simulink model "RELY_PT_Simscape_model_clean"  (R2023b)
settings: Solver=VariableStepAuto  StartTime=0.0  StopTime=90  RelTol=1e-3
PreLoadFcn:
  | %warning('off', 'physmod:simscape:engine:sli:zc:ZeroCrossingsGloballyOff');
  | %warning('off', 'SimulinkExecution:DE:MinStepSizeForDAEWarning');
  | %warning('off')
StopFcn:
  | [lastWarningMessage, warningId] = lastwarn
  | display(lastwarn)
model workspace (MAT data in the model file):
  H_n0_a0 = 0
  H_n0_a12 = 0
  H_n0_a18 = 0
  H_n0_a24 = 0
  H_n0_a3 = 0
  H_n0_a30 = 0
  H_n0_a6 = 0
  H_n1000_a0 = 41.890778
  H_n1000_a12 = [39.720451 39.531112 38.954187 38.409379 37.371519 36.969249 36.145323 35.016504 34.41791 32.725714 29.62353 26.475564 ... (14 elements, 14x1)]
  H_n1000_a18 = [40.963701 39.338792 38.382958 37.856819 36.842644 36.842643 36.420949 35.987956 35.163037 34.563355 33.765342 32.552991 ... (15 elements, 15x1)]
  H_n1000_a24 = [38.981139 38.080649 37.518525 37.024422 36.538756 36.021688 35.445183 35.316271 34.435388 33.472576 31.549447 29.78877 ... (14 elements, 14x1)]
  H_n1000_a3 = [41.890778; 40.628119; 36.670096; 26.463116; 15.07804; 14.630001]
  H_n1000_a30 = [38.909304 37.733775 37.005538 36.587968 36.205827 35.762706 35.340739 35.100753 34.52749 33.838404 32.675216 31.34989 ... (15 elements, 15x1)]
  H_n1000_a6 = [40.993428; 40.166943; 39.662948; 38.765772; 36.424758; 29.65575; 24.303713; 16.252806]
  H_n200_a0 = 3.238104
  H_n200_a12 = [1.067777; 1.033602; 0.921547; 0.765236; 0.326687]
  H_n200_a18 = [2.311027; 0.686118; 0]
  H_n200_a24 = [0.328465; 0]
  H_n200_a3 = [3.238104; 1.975445; 0]
  H_n200_a30 = [0.25663; 0]
  H_n200_a6 = [2.340754; 1.514269; 1.010274; 0.113098; 0]
  H_n300_a0 = 5.257449
  H_n300_a12 = [3.087122; 2.979731; 2.862074; 2.645072; 2.104165; 1.313568; 0.689971; 0.506891]
  H_n300_a18 = [4.330372; 2.705463; 1.749629; 1.22349; 0.209315; 0.209314; 0]
  H_n300_a24 = [2.34781; 1.44732; 0.885196; 0.391093; 0]
  H_n300_a3 = [5.257449; 3.99479; 0.036767; 0]
  H_n300_a30 = [2.275975; 1.100446; 0.372209; 0]
  H_n300_a6 = [4.360099; 3.533614; 3.029619; 2.132443; 0]
  H_n400_a0 = 8.103137
  H_n400_a12 = [5.93281; 5.819804; 5.646321; 5.369927; 5.096687; 4.506441; 3.638024; 2.520335; 1.315366]
  H_n400_a18 = [7.17606; 5.551151; 4.595317; 4.069178; 3.055003; 3.055002; 2.633308; 2.200315; 1.375396; 0.775714; 0]
  H_n400_a24 = [5.193498; 4.293008; 3.730884; 3.236781; 2.751115; 2.234047; 1.657542; 1.52863; 0.647747; 0]
  H_n400_a3 = [8.103137; 6.840478; 2.882455; 0]
  H_n400_a30 = [5.121663; 3.946134; 3.217897; 2.800327; 2.418186; 1.975065; 1.553098; 1.313112; 0.739849; 0.050763; 0]
  H_n400_a6 = [7.205787; 6.379302; 5.875307; 4.978131; 2.637117; 0]
  H_n500_a0 = 11.717619
  H_n500_a12 = [9.547292; 9.47316; 9.245124; 8.930514; 8.600563; 8.213538; 7.488479; 5.941616; 4.256148; 2.697226; 2.352739]
  H_n500_a18 = [10.790542 9.165633 8.209799 7.68366 6.669485 6.669484 6.24779 5.814797 4.989878 4.390196 3.592183 2.379832 ... (14 elements, 14x1)]
  H_n500_a24 = [8.80798; 7.90749; 7.345366; 6.851263; 6.365597; 5.848529; 5.272024; 5.143112; 4.262229; 3.299417; 1.376288; 0]
  H_n500_a3 = [11.717619; 10.45496; 6.496937; 0]
  H_n500_a30 = [8.736145 7.560616 6.832379 6.414809 6.032668 5.589547 5.16758 4.927594 4.354331 3.665245 2.502057 1.176731 ... (13 elements, 13x1)]
  H_n500_a6 = [10.820269; 9.993784; 9.489789; 8.592613; 6.251599; 0]
  H_n600_a0 = 16.132839
  H_n600_a12 = [13.962512; 13.826181; 13.39772; 12.968961; 12.407512; 11.706692; 10.267649; 7.799717; 4.805174; 3.660927]
  H_n600_a18 = [15.205762 13.580853 12.625019 12.09888 11.084705 11.084704 10.66301 10.230017 9.405098 8.805416 8.007403 6.795052 ... (15 elements, 15x1)]
  H_n600_a24 = [13.2232 12.32271 11.760586 11.266483 10.780817 10.263749 9.687244 9.558332 8.677449 7.714637 5.791508 4.030831 ... (14 elements, 14x1)]
  H_n600_a3 = [16.132839; 14.87018; 10.912157; 0.705177; 0]
  H_n600_a30 = [13.151365 11.975836 11.247599 10.830029 10.447888 10.004767 9.5828 9.342814 8.769551 8.080465 6.917277 5.591951 ... (15 elements, 15x1)]
  H_n600_a6 = [15.235489; 14.409004; 13.905009; 13.007833; 10.666819; 3.897811; 0]
  H_n800_a0 = 27.361581
  H_n800_a12 = [25.191254 25.111402 24.820598 24.424515 23.864287 23.409359 22.670967 21.888411 20.849925 19.271611 15.931711 12.191149 ... (13 elements, 13x1)]
  H_n800_a18 = [26.434504 24.809595 23.853761 23.327622 22.313447 22.313446 21.891752 21.458759 20.63384 20.034158 19.236145 18.023794 ... (15 elements, 15x1)]
  H_n800_a24 = [24.451942 23.551452 22.989328 22.495225 22.009559 21.492491 20.915986 20.787074 19.906191 18.943379 17.02025 15.259573 ... (14 elements, 14x1)]
  H_n800_a3 = [27.361581; 26.098922; 22.140899; 11.933919; 0.548843; 0.100804]
  H_n800_a30 = [24.380107 23.204578 22.476341 22.058771 21.67663 21.233509 20.811542 20.571556 19.998293 19.309207 18.146019 16.820693 ... (15 elements, 15x1)]
  H_n800_a6 = [26.464231; 25.637746; 25.133751; 24.236575; 21.895561; 15.126553; 9.774516; 1.723609]
  Q_n0_a0 = 0
  Q_n0_a12 = 0
  Q_n0_a18 = 0
  Q_n0_a24 = 0
  Q_n0_a3 = 0
  Q_n0_a30 = 0
  Q_n0_a6 = 0
  Q_n1000_a0 = 0
  Q_n1000_a12 = [1.414248 19.568281 42.238315 63.498226 84.388459 102.222447 118.464783 143.286635 161.301465 179.936079 204.714875 220.907445 ... (14 elements, 14x1)]
  Q_n1000_a18 = [1.408805 18.494853 42.193847 62.613149 82.187881 100.830014 121.754975 143.135578 163.193197 178.395322 191.000248 206.658481 ... (15 elements, 15x1)]
  Q_n1000_a24 = [1.423901 19.712366 41.694896 61.712178 79.84989 98.707828 119.980398 158.480134 182.365548 200.814664 230.378522 251.54405 ... (14 elements, 14x1)]
  Q_n1000_a3 = [1.421904; 19.241198; 41.163866; 59.088119; 65.74439; 65.877885]
  Q_n1000_a30 = [1.416544 19.140809 40.908666 60.206263 78.832144 103.65752 124.537322 147.320333 173.202338 192.924112 213.836687 234.126658 ... (15 elements, 15x1)]
  Q_n1000_a6 = [1.391187; 19.624304; 38.811559; 58.375933; 80.275679; 102.989156; 113.538726; 121.386064]
  Q_n200_a0 = 0
  Q_n200_a12 = [1.34007; 7.497876; 25.362531; 37.225803; 48.080824]
  Q_n200_a18 = [1.408805; 18.494853; 42.193847]
  Q_n200_a24 = [1.423901; 19.712366]
  Q_n200_a3 = [1.421904; 19.241198; 41.163866]
  Q_n200_a30 = [1.416544; 19.140809]
  Q_n200_a6 = [1.391187; 19.624304; 38.811559; 58.375933; 80.275679]
  Q_n300_a0 = 0
  Q_n300_a12 = [1.367844; 15.571876; 31.1207; 46.669706; 61.781875; 72.981285; 80.669073; 83.063222]
  Q_n300_a18 = [1.408805; 18.494853; 42.193847; 62.613149; 82.187881; 100.830014; 121.754975]
  Q_n300_a24 = [1.423901; 19.712366; 41.694896; 61.712178; 79.84989]
  Q_n300_a3 = [1.421904; 19.241198; 41.163866; 59.088119]
  Q_n300_a30 = [1.416544; 19.140809; 40.908666; 60.206263]
  Q_n300_a6 = [1.391187; 19.624304; 38.811559; 58.375933; 80.275679]
  Q_n400_a0 = 0
  Q_n400_a12 = [1.344743; 14.017933; 27.304134; 46.234876; 61.473368; 76.555174; 87.737013; 99.497539; 110.117964]
  Q_n400_a18 = [1.408805; 18.494853; 42.193847; 62.613149; 82.187881; 100.830014; 121.754975; 143.135578; 163.193197; 178.395322; 191.000248]
  Q_n400_a24 = [1.423901; 19.712366; 41.694896; 61.712178; 79.84989; 98.707828; 119.980398; 158.480134; 182.365548; 200.814664]
  Q_n400_a3 = [1.421904; 19.241198; 41.163866; 59.088119]
  Q_n400_a30 = [1.416544; 19.140809; 40.908666; 60.206263; 78.832144; 103.65752; 124.537322; 147.320333; 173.202338; 192.924112; 213.836687]
  Q_n400_a6 = [1.391187; 19.624304; 38.811559; 58.375933; 80.275679; 102.989156]
  Q_n500_a0 = 0
  Q_n500_a12 = [1.413707; 13.380401; 28.647003; 44.528782; 60.801181; 80.900847; 92.946609; 109.551251; 123.738046; 134.385391; 136.883854]
  Q_n500_a18 = [1.408805 18.494853 42.193847 62.613149 82.187881 100.830014 121.754975 143.135578 163.193197 178.395322 191.000248 206.658481 ... (14 elements, 14x1)]
  Q_n500_a24 = [1.423901; 19.712366; 41.694896; 61.712178; 79.84989; 98.707828; 119.980398; 158.480134; 182.365548; 200.814664; 230.378522; 251.54405]
  Q_n500_a3 = [1.421904; 19.241198; 41.163866; 59.088119]
  Q_n500_a30 = [1.416544 19.140809 40.908666 60.206263 78.832144 103.65752 124.537322 147.320333 173.202338 192.924112 213.836687 234.126658 ... (13 elements, 13x1)]
  Q_n500_a6 = [1.391187; 19.624304; 38.811559; 58.375933; 80.275679; 102.989156]
  Q_n600_a0 = 0
  Q_n600_a12 = [1.382688; 19.531879; 40.922311; 61.362127; 81.302459; 103.019269; 120.607387; 139.781266; 159.674546; 165.725558]
  Q_n600_a18 = [1.408805 18.494853 42.193847 62.613149 82.187881 100.830014 121.754975 143.135578 163.193197 178.395322 191.000248 206.658481 ... (15 elements, 15x1)]
  Q_n600_a24 = [1.423901 19.712366 41.694896 61.712178 79.84989 98.707828 119.980398 158.480134 182.365548 200.814664 230.378522 251.54405 ... (14 elements, 14x1)]
  Q_n600_a3 = [1.421904; 19.241198; 41.163866; 59.088119; 65.74439]
  Q_n600_a30 = [1.416544 19.140809 40.908666 60.206263 78.832144 103.65752 124.537322 147.320333 173.202338 192.924112 213.836687 234.126658 ... (15 elements, 15x1)]
  Q_n600_a6 = [1.391187; 19.624304; 38.811559; 58.375933; 80.275679; 102.989156; 113.538726]
  Q_n800_a0 = 0
  Q_n800_a12 = [1.454137 13.240478 29.958658 46.304107 64.130487 81.966165 101.000644 121.860549 141.622312 158.000863 181.468089 200.017812 ... (13 elements, 13x1)]
  Q_n800_a18 = [1.408805 18.494853 42.193847 62.613149 82.187881 100.830014 121.754975 143.135578 163.193197 178.395322 191.000248 206.658481 ... (15 elements, 15x1)]
  Q_n800_a24 = [1.423901 19.712366 41.694896 61.712178 79.84989 98.707828 119.980398 158.480134 182.365548 200.814664 230.378522 251.54405 ... (14 elements, 14x1)]
  Q_n800_a3 = [1.421904; 19.241198; 41.163866; 59.088119; 65.74439; 65.877885]
  Q_n800_a30 = [1.416544 19.140809 40.908666 60.206263 78.832144 103.65752 124.537322 147.320333 173.202338 192.924112 213.836687 234.126658 ... (15 elements, 15x1)]
  Q_n800_a6 = [1.391187; 19.624304; 38.811559; 58.375933; 80.275679; 102.989156; 113.538726; 121.386064]
  Qt_n0_a0 = 0
  Qt_n0_a12 = 0
  Qt_n0_a18 = 0
  Qt_n0_a24 = 0
  Qt_n0_a3 = 0
  Qt_n0_a30 = 0
  Qt_n0_a6 = 0
  Qt_n1000_a0 = 0
  Qt_n1000_a12 = [0 16.7063426923 33.4126853846 50.1190280769 66.8253707692 83.5317134615 100.238056154 116.944398846 133.650741538 150.357084231 167.063426923 183.769769615 ... (14 elements, 14x1)]
  Qt_n1000_a18 = [0 19.1696658462 38.3393316923 57.5089975385 76.6786633846 95.8483292308 115.017995077 134.187660923 153.357326769 172.526992615 191.696658462 210.866324308 ... (14 elements, 14x1)]
  Qt_n1000_a24 = [0 21.8796540769 43.7593081538 65.6389622308 87.5186163077 109.398270385 131.277924462 153.157578538 175.037232615 196.916886692 218.796540769 240.676194846 ... (14 elements, 14x1)]
  Qt_n1000_a3 = [0 5.06752961538 10.1350592308 15.2025888462 20.2701184615 25.3376480769 30.4051776923 35.4727073077 40.5402369231 45.6077665385 50.6752961538 55.7428257692 ... (14 elements, 14x1)]
  Qt_n1000_a30 = [0 22.2052569231 44.4105138462 66.6157707692 88.8210276923 111.026284615 133.231541538 155.436798462 177.642055385 199.847312308 222.052569231 244.257826154 ... (14 elements, 14x1)]
  Qt_n1000_a6 = [0 9.33738953846 18.6747790769 28.0121686154 37.3495581538 46.6869476923 56.0243372308 65.3617267692 74.6991163077 84.0365058462 93.3738953846 102.711284923 ... (14 elements, 14x1)]
  Qt_n200_a0 = 0
  Qt_n200_a12 = [0; 54.29561375; 108.5912275; 162.88684125; 217.182455]
  Qt_n200_a18 = [0; 62.301414; 124.602828; 186.904242; 249.205656]
  Qt_n200_a24 = [0; 71.10887575; 142.2177515; 213.32662725; 284.435503]
  Qt_n200_a3 = [0; 16.46947125; 32.9389425; 49.40841375; 65.877885]
  Qt_n200_a30 = [0; 72.167085; 144.33417; 216.501255; 288.66834]
  Qt_n200_a6 = [0; 30.346516; 60.693032; 91.039548; 121.386064]
  Qt_n300_a0 = 0
  Qt_n300_a12 = [0; 31.026065; 62.05213; 93.078195; 124.10426; 155.130325; 186.15639; 217.182455]
  Qt_n300_a18 = [0; 35.600808; 71.201616; 106.802424; 142.403232; 178.00404; 213.604848; 249.205656]
  Qt_n300_a24 = [0; 40.6336432857; 81.2672865714; 121.900929857; 162.534573143; 203.168216429; 243.801859714; 284.435503]
  Qt_n300_a3 = [0; 9.41112642857; 18.8222528571; 28.2333792857; 37.6445057143; 47.0556321429; 56.4667585714; 65.877885]
  Qt_n300_a30 = [0; 41.2383342857; 82.4766685714; 123.715002857; 164.953337143; 206.191671429; 247.430005714; 288.66834]
  Qt_n300_a6 = [0; 17.3408662857; 34.6817325714; 52.0225988571; 69.3634651429; 86.7043314286; 104.045197714; 121.386064]
  Qt_n400_a0 = 0
  Qt_n400_a12 = [0; 27.147806875; 54.29561375; 81.443420625; 108.5912275; 135.739034375; 162.88684125; 190.034648125; 217.182455]
  Qt_n400_a18 = [0; 31.150707; 62.301414; 93.452121; 124.602828; 155.753535; 186.904242; 218.054949; 249.205656]
  Qt_n400_a24 = [0; 35.554437875; 71.10887575; 106.663313625; 142.2177515; 177.772189375; 213.32662725; 248.881065125; 284.435503]
  Qt_n400_a3 = [0; 8.234735625; 16.46947125; 24.704206875; 32.9389425; 41.173678125; 49.40841375; 57.643149375; 65.877885]
  Qt_n400_a30 = [0; 36.0835425; 72.167085; 108.2506275; 144.33417; 180.4177125; 216.501255; 252.5847975; 288.66834]
  Qt_n400_a6 = [0; 15.173258; 30.346516; 45.519774; 60.693032; 75.86629; 91.039548; 106.212806; 121.386064]
  Qt_n500_a0 = 0
  Qt_n500_a12 = [0; 21.7182455; 43.436491; 65.1547365; 86.872982; 108.5912275; 130.309473; 152.0277185; 173.745964; 195.4642095; 217.182455]
  Qt_n500_a18 = [0; 24.9205656; 49.8411312; 74.7616968; 99.6822624; 124.602828; 149.5233936; 174.4439592; 199.3645248; 224.2850904; 249.205656]
  Qt_n500_a24 = [0; 28.4435503; 56.8871006; 85.3306509; 113.7742012; 142.2177515; 170.6613018; 199.1048521; 227.5484024; 255.9919527; 284.435503]
  Qt_n500_a3 = [0; 6.5877885; 13.175577; 19.7633655; 26.351154; 32.9389425; 39.526731; 46.1145195; 52.702308; 59.2900965; 65.877885]
  Qt_n500_a30 = [0; 28.866834; 57.733668; 86.600502; 115.467336; 144.33417; 173.201004; 202.067838; 230.934672; 259.801506; 288.66834]
  Qt_n500_a6 = [0; 12.1386064; 24.2772128; 36.4158192; 48.5544256; 60.693032; 72.8316384; 84.9702448; 97.1088512; 109.2474576; 121.386064]
  Qt_n600_a0 = 0
  Qt_n600_a12 = [0; 24.1313838889; 48.2627677778; 72.3941516667; 96.5255355556; 120.656919444; 144.788303333; 168.919687222; 193.051071111; 217.182455]
  Qt_n600_a18 = [0; 27.6895173333; 55.3790346667; 83.068552; 110.758069333; 138.447586667; 166.137104; 193.826621333; 221.516138667; 249.205656]
  Qt_n600_a24 = [0; 31.6039447778; 63.2078895556; 94.8118343333; 126.415779111; 158.019723889; 189.623668667; 221.227613444; 252.831558222; 284.435503]
  Qt_n600_a3 = [0; 7.319765; 14.63953; 21.959295; 29.27906; 36.598825; 43.91859; 51.238355; 58.55812; 65.877885]
  Qt_n600_a30 = [0; 32.07426; 64.14852; 96.22278; 128.29704; 160.3713; 192.44556; 224.51982; 256.59408; 288.66834]
  Qt_n600_a6 = [0; 13.4873404444; 26.9746808889; 40.4620213333; 53.9493617778; 67.4367022222; 80.9240426667; 94.4113831111; 107.898723556; 121.386064]
  Qt_n800_a0 = 0
  Qt_n800_a12 = [1.454137 13.240478 29.958658 46.304107 64.130487 81.966165 101.000644 121.860549 141.622312 158.000863 181.468089 200.017812 ... (13 elements, 13x1)]
  Qt_n800_a18 = [1.408805 18.494853 42.193847 62.613149 82.187881 100.830014 121.754975 143.135578 163.193197 178.395322 191.000248 206.658481 ... (15 elements, 15x1)]
  Qt_n800_a24 = [1.423901 19.712366 41.694896 61.712178 79.84989 98.707828 119.980398 158.480134 182.365548 200.814664 230.378522 251.54405 ... (14 elements, 14x1)]
  Qt_n800_a3 = [1.421904; 19.241198; 41.163866; 59.088119; 65.74439; 65.877885]
  Qt_n800_a30 = [1.416544 19.140809 40.908666 60.206263 78.832144 103.65752 124.537322 147.320333 173.202338 192.924112 213.836687 234.126658 ... (15 elements, 15x1)]
  Qt_n800_a6 = [1.391187; 19.624304; 38.811559; 58.375933; 80.275679; 102.989156; 113.538726; 121.386064]
  T_n0_a0 = 0
  T_n0_a12 = 0
  T_n0_a18 = 0
  T_n0_a24 = 0
  T_n0_a3 = 0
  T_n0_a30 = 0
  T_n0_a6 = 0
  T_n1000_a0 = 212.918607715
  T_n1000_a12 = [277.00328 303.197846 359.332799 415.990553 473.006501 524.971962 568.439998 614.751636 645.453671 686.416528 736.459699 766.00495 ... (14 elements, 14x1)]
  T_n1000_a18 = [404.787518585 404.787519585 404.787520585 452.001035443 510.769182758 569.170823248 619.258390544 671.193440572 702.288039208 740.090455903 784.6835679 804.130666851 ... (14 elements, 14x1)]
  T_n1000_a24 = [392.733848002 392.733849002 439.832412682 496.757162262 558.754412487 616.785919809 664.650726048 714.600674645 742.820149063 778.056363106 818.81453792 829.567277535 ... (14 elements, 14x1)]
  T_n1000_a3 = [212.918607715 212.918608715 228.059187273 245.258629322 263.444651993 280.537619561 295.489881395 314.864010802 328.777823048 350.303733023 379.296474597 399.333660461 ... (14 elements, 14x1)]
  T_n1000_a30 = [421.41608902 421.41609002 440.120958305 494.847705165 558.496053897 619.777761537 670.689767338 722.468413619 750.521719432 783.871432441 821.31664772 828.125692716 ... (14 elements, 14x1)]
  T_n1000_a6 = [230.781502838 242.11861906 275.591838884 308.353632665 342.191487589 374.384720871 403.309826474 437.782449643 463.92378222 499.743176352 544.837963229 574.949829916 ... (14 elements, 14x1)]
  T_n200_a0 = 11.7025560582
  T_n200_a12 = [15.224815; 17.437209; 27.286419; 32.75526; 36.736891]
  T_n200_a18 = [22.2481664649; 22.2481674649; 29.7967404674; 35.0029856064; 37.9298346396]
  T_n200_a24 = [21.5856656285; 21.5856666285; 31.8450559685; 36.603000066; 37.244980588]
  T_n200_a3 = [11.7025560582; 11.7025570582; 14.0701061615; 16.8185305371; 19.8004114128]
  T_n200_a30 = [23.1621156015; 23.1621166015; 32.1752703252; 36.7584990128; 37.0567955811]
  T_n200_a6 = [12.6843468645; 12.8324608472; 19.3918858683; 24.1271526112; 28.1688483977]
  T_n300_a0 = 21.9563918625
  T_n300_a12 = [28.564871; 37.811393; 51.060297; 62.173487; 71.550804; 76.450124; 78.444822; 79.17734]
  T_n300_a18 = [41.7421167388; 42.9108918828; 55.1360860791; 67.6540960449; 78.0129967452; 82.131335262; 82.2106920633; 82.2106930633]
  T_n300_a24 = [40.4991294887; 46.5570500429; 60.4440800927; 72.9025088968; 82.8132330772; 86.1815876807; 86.1815886807; 86.1815896807]
  T_n300_a3 = [21.9563918625; 24.2987024018; 28.8525912211; 32.6741136324; 36.5007981988; 39.0750608961; 40.992116131; 42.6749206015]
  T_n300_a30 = [43.4568724969; 46.6716879727; 60.3340767989; 73.4500908753; 83.7275835225; 86.7267109875; 86.7267119875; 86.7267129875]
  T_n300_a6 = [23.798432487; 29.1774180928; 37.1526626527; 44.1911964018; 51.0954995027; 55.8783235655; 59.0146995211; 60.7110298744]
  T_n400_a0 = 36.5747783831
  T_n400_a12 = [47.583129; 57.587133; 70.997483; 92.596133; 105.648342; 118.067856; 125.504464; 132.006944; 135.802681]
  T_n400_a18 = [69.533677415; 69.533678415; 76.8740175836; 100.303252833; 115.367876869; 128.336169471; 134.116808932; 137.955920328; 140.212551845]
  T_n400_a24 = [67.4631193976; 71.5608625438; 84.4618055352; 108.830263209; 123.298603747; 135.640440023; 140.247395505; 141.469481676; 141.469482676]
  T_n400_a3 = [36.5747783831; 37.7251893206; 41.1960296213; 49.6890098491; 54.4770417739; 60.123752896; 64.4415785534; 69.2427899981; 73.1947881697]
  T_n400_a30 = [72.390103563; 72.390104563; 84.1709945503; 109.287902187; 124.577137193; 137.012881865; 140.843202467; 141.001174713; 141.001175713]
  T_n400_a6 = [39.6432346229; 44.8168070482; 52.2487527018; 66.1049603064; 75.082061528; 84.972188629; 92.4451631986; 99.6500611017; 104.129800562]
  T_n500_a0 = 54.638111826
  T_n500_a12 = [71.083201; 82.173064; 102.133248; 124.085102; 147.054333; 166.819409; 179.223177; 194.174843; 204.809839; 209.250296; 210.496478]
  T_n500_a18 = [103.874555369; 103.874556369; 111.971411057; 133.975134134; 159.674103654; 182.16661684; 195.237724451; 209.113945989; 216.990100397; 217.817160263; 217.817161263]
  T_n500_a24 = [100.781402506; 103.745756337; 122.884743199; 146.67783451; 172.687108198; 194.6892854; 206.759491412; 219.699188786; 225.542233105; 225.542234105; 225.542235105]
  T_n500_a3 = [54.638111826; 55.3756440027; 61.8869149757; 69.4496573087; 78.1013520092; 86.0195980434; 91.3358717102; 99.1482056914; 105.978124691; 110.324399881; 113.453173415]
  T_n500_a30 = [108.14169623; 108.14169723; 122.461015878; 146.537256202; 173.69605955; 196.708097903; 208.970369715; 221.255795744; 225.791005625; 225.791006625; 225.791007625]
  T_n500_a6 = [59.2219989356; 64.7472437047; 76.6568548901; 89.9397391904; 104.73390719; 118.55505627; 128.538611573; 141.568983951; 152.461177958; 158.612181364; 161.402971662]
  T_n600_a0 = 76.867003996
  T_n600_a12 = [100.00259; 121.04164; 155.003179; 190.565914; 219.357637; 243.674297; 266.051748; 283.258948; 297.465728; 299.083675]
  T_n600_a18 = [146.134732622; 146.134733622; 168.784930149; 205.972762496; 238.873142197; 265.77258359; 287.747983451; 301.365627068; 310.186180583; 310.186181583]
  T_n600_a24 = [141.78316582; 151.644017044; 185.472115884; 224.665102596; 256.903171302; 282.518160305; 303.137003848; 314.154023247; 317.032846233; 317.032847233]
  T_n600_a3 = [76.867003996; 80.5184824525; 92.0750202273; 104.524650538; 114.657143003; 124.465033252; 135.526566037; 146.079378975; 156.481270539; 161.199808984]
  T_n600_a30 = [152.137911037; 153.157263195; 184.752954542; 224.955132121; 259.040760261; 285.649929708; 305.759721542; 314.944478723; 315.773465036; 315.773466036]
  T_n600_a6 = [83.3157932567; 94.825703277; 115.297380604; 137.074433445; 155.769374031; 173.678780092; 192.721213139; 209.938294249; 225.088940119; 229.32922384]
  T_n800_a0 = 134.014292
  T_n800_a12 = [177.472657 191.031966 222.274404 256.025382 295.517459 337.418928 374.986676 405.355521 436.442001 464.646182 498.675007 515.239787 ... (13 elements, 13x1)]
  T_n800_a18 = [258.973744 258.973745 261.725534 300.744533 341.164912 384.371738 411.583185 443.99362 474.009937 494.394349 508.380623 522.912901 ... (15 elements, 15x1)]
  T_n800_a24 = [249.324679 250.177033 276.500869 309.026906 346.334209 381.490782 412.86896 468.224431 499.703761 515.781407 537.873966 541.192558 ... (14 elements, 14x1)]
  T_n800_a3 = [134.014292; 165.189551; 220.071093; 267.680146; 284.992769; 285.510636]
  T_n800_a30 = [268.511256 268.511257 272.073856 305.537173 345.09648 390.152116 420.857847 452.358387 489.729128 512.267985 526.708091 538.084495 ... (15 elements, 15x1)]
  T_n800_a6 = [145.892985; 179.168033; 221.533717; 266.922578; 322.43552; 373.367837; 392.8052; 406.386096]
  a_Spalt = 0.0001
  a_max = 0.034
  final_flow_rate = 0.2
  g = 9.81
  h_ausgebl = 0.32549
  h_min = 0.2
  h_voll = 0.465
  input : object (value not decoded)
  max_volume = 0.06
  mdl = 'RELY_PT_Simscape_model_clean'
  out : Simulink.SimulationOutput (value not decoded)
  p_air = 4
  rho_water = 997
  sync_speed = 850
libraries: fl_lib x23, nesl_utility x12, SimscapeFluids_lib x8, simulink x5, simulink_gym x2
(part 4 of 4)

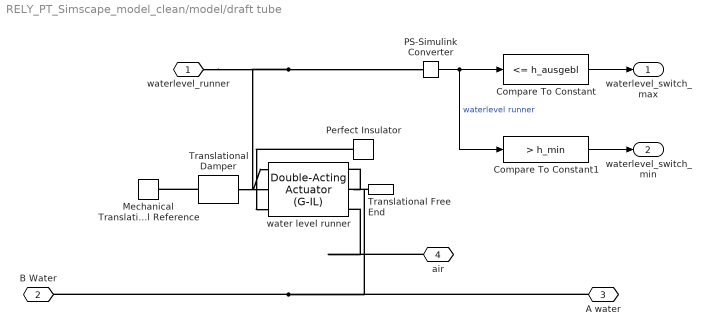
== system RELY_PT_Simscape_model_clean/model/draft tube ==
  Compare To Constant : simulink/Logic and Bit Operations/Compare To Constant  relop=<=  const=h_ausgebl  OutDataTypeStr=boolean
  Compare To Constant1 : simulink/Logic and Bit Operations/Compare To Constant  relop=>  const=h_min  OutDataTypeStr=boolean
  Mechanical Translational Reference : fl_lib/Mechanical/Translational Elements/Mechanical Translational Reference
  PS-Simulink Converter : nesl_utility/PS-Simulink Converter  PhysicalDomain=network_engine_domain  SubClassName=ps_output  LeftPortType=input  RightPortType=output  PseudoPeriodic=off  Frequencies=[]  VectorFormat=inherit  Unit=m  AffineConversion=off
  Perfect Insulator : fl_lib/Thermal/Thermal Elements/Perfect Insulator  T_specify=off  T_priority=None  T=0 K  T_nominal_specify=off  T_nominal_unit=K  T_nominal_value=1
  Translational Damper : fl_lib/Mechanical/Translational Elements/Translational Damper  D=100 N*s/m  v_specify=off  v_priority=None  v=0 m/s  v_nominal_specify=off  v_nominal_unit=m/s  v_nominal_value=1  f_specify=off  f_priority=None  f=0 N  f_nominal_specify=off  f_nominal_unit=N  f_nominal_value=1
  Translational Free End : fl_lib/Mechanical/Translational Elements/Translational Free End  v_specify=off  v_priority=None  v=0 m/s  v_nominal_specify=off  v_nominal_unit=m/s  v_nominal_value=1
      settings: InternalSimscapePortConfiguration="{\"Bottom\":[],\"Left\":[{\"id\":\"V\",\"label\":\"\",\"type\":\"foundation.mechanical.translational.translational\"}],\"Right\":[],\"Top\":[]}"
  water level runner : SimscapeFluids_lib/Fluid Network Interfaces/Actuators/Double-Acting Actuator (G-IL)  mech_orientation=foundation.enum.MechOrientationTranslational.Positive  stroke=h_voll m  x0=h_voll m  hardstop_model=simscape.enum.hardstop.smooth  stiff_coeff=1e10 N/m  damping_coeff=15000 N/(m/s)  transition=0.1 mm  coeff_rest=0.7  v_tol=0.001 m/s  f_tol=0.001 N  piston_area_A=0.1 m^2  dead_volume_A=1e-5 m^3  dynamic_compressibility=false  p0_A=1 bar  environment_spec_A=foundation.enum.pressure_spec.atmospheric  environment_p_A=0.101325 MPa  piston_area_B=0.1 m^2  area_B=1.131e-4 m^2  dead_volume_B=1e-5 m^3  p0_B=0.101324 MPa  T0_B=290 K  environment_spec_B=foundation.enum.pressure_spec.atmospheric  environment_p_B=p_atm Pa
      settings: InternalSimscapePortConfiguration="{\"Bottom\":[{\"id\":\"A\",\"label\":\"A\",\"type\":\"foundation.isothermal_liquid.isothermal_liquid\"},{\"id\":\"B\",\"label\":\"B\",\"type\":\"foundation.gas.gas\"}],\"Left\":[{\"id\":\"C\",\"label\":\"C\",\"type\":\"foundation.mechanical.translational.translational\"}],\"Right\":[{\"id\":\"R\",\"label\":\"R\",\"type\":\"foundation.mechanical.translational.translational\"}],\"Top\":[{\"id\":\"p_out\",\"label\":\"p\",\"type\":\"output\"},{\"id\":\"H\",\"label\":\"H\",\"type\":\"foundation.thermal.thermal\"}]}"
  waterlevel_runner : PMIOPort  Side=Left
  B Water : PMIOPort  Port=2  Side=Left
  A water : PMIOPort  Port=3  Side=Left
  air : PMIOPort  Port=4  Side=Right
  waterlevel_switch_max : Outport
  waterlevel_switch_min : Outport  Port=2
  wires:
  Compare To Constant/1 -> waterlevel_switch_max/1
  Compare To Constant1/1 -> waterlevel_switch_min/1
  PS-Simulink Converter/1 -> Compare To Constant1/1, Compare To Constant/1  "waterlevel runner"
  connections:
  Translational Damper/LConn1 -- water level runner/LConn1
  Perfect Insulator/LConn1 -- water level runner/LConn3
  air/RConn1 -- water level runner/RConn3
  waterlevel_runner/RConn1 -- water level runner/LConn2 -- PS-Simulink Converter/LConn1
  Translational Damper/RConn1 -- Mechanical Translational Reference/LConn1
  Translational Free End/LConn1 -- water level runner/RConn1
  A water/RConn1 -- B Water/RConn1 -- water level runner/RConn2

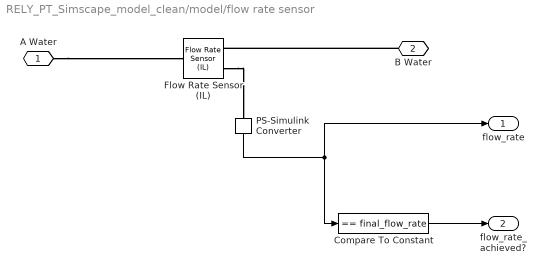
== system RELY_PT_Simscape_model_clean/model/flow rate sensor ==
  Compare To Constant : simulink/Logic and Bit Operations/Compare To Constant  relop===  const=final_flow_rate  OutDataTypeStr=boolean
  Flow Rate Sensor (IL) : fl_lib/Isothermal Liquid/Sensors/Flow Rate Sensor (IL)  sensor_type=foundation.enum.mass_volumetric_sensor.volumetric
      settings: InternalSimscapePortConfiguration="{\"Bottom\":[],\"Left\":[{\"id\":\"A\",\"label\":\"A\",\"type\":\"foundation.isothermal_liquid.isothermal_liquid\"}],\"Right\":[{\"id\":\"B\",\"label\":\"B\",\"type\":\"foundation.isothermal_liquid.isothermal_liquid\"},{\"id\":\"V\",\"label\":\"V\",\"type\":\"output\"}],\"Top\":[]}"
  PS-Simulink Converter : nesl_utility/PS-Simulink Converter  PhysicalDomain=network_engine_domain  SubClassName=ps_output  LeftPortType=input  RightPortType=output  PseudoPeriodic=off  Frequencies=[]  VectorFormat=inherit  Unit=m^3/s  AffineConversion=off
  A Water : PMIOPort  Side=Left
  B Water : PMIOPort  Port=2  Side=Right
  flow_rate : Outport
  flow_rate_achieved? : Outport  Port=2
  wires:
  PS-Simulink Converter/1 -> Compare To Constant/1, flow_rate/1
  Compare To Constant/1 -> flow_rate_achieved?/1
  connections:
  B Water/RConn1 -- Flow Rate Sensor (IL)/RConn1
  Flow Rate Sensor (IL)/RConn2 -- PS-Simulink Converter/LConn1
  A Water/RConn1 -- Flow Rate Sensor (IL)/LConn1

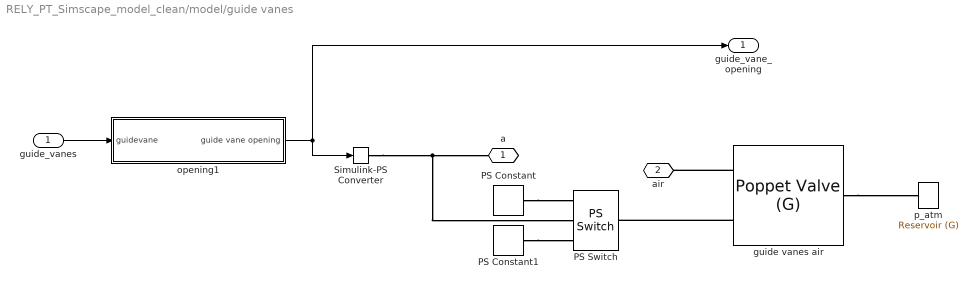
== system RELY_PT_Simscape_model_clean/model/guide vanes ==
  guide_vanes : Inport
  PS Constant : fl_lib/Physical Signals/Sources/PS Constant  constant=1
  PS Constant1 : fl_lib/Physical Signals/Sources/PS Constant  constant=0.0000001
  PS Switch : fl_lib/Physical Signals/Nonlinear Operators/PS Switch  Threshold=0.001 m
      settings: InternalSimscapePortConfiguration="{\"Bottom\":[],\"Left\":[{\"id\":\"I1\",\"label\":\"\",\"type\":\"input\"},{\"id\":\"I2\",\"label\":\"\",\"type\":\"input\"},{\"id\":\"I3\",\"label\":\"\",\"type\":\"input\"}],\"Right\":[{\"id\":\"O\",\"label\":\"\",\"type\":\"output\"}],\"Top\":[]}"
  Simulink-PS Converter : nesl_utility/Simulink-PS Converter  PhysicalDomain=network_engine_domain  SubClassName=ps_input  LeftPortType=input  RightPortType=output  PseudoPeriodic=off  Frequencies=[]  NoiseDistribution=none  NoiseParameters=[]  Unit=m  AffineConversion=off  FilteringAndDerivatives=provide  SimscapeFilterOrder=1  InputFilterTimeConstant=0.001  UdotUserProvided=0
  guide vanes air : SimscapeFluids_lib/Gas/Valves & Orifices/Flow Control Valves/Poppet Valve (G)  valve_seat_geometry=fluids.gas.valves_orifices.flow_control_valves.enum.ValveSeatGeometry.Conical  cone_angle=120 deg  diam_ball=0.015 m  diam_orifice=0.003 m  valve_parameterization=fluids.gas.valves_orifices.flow_control_valves.enum.OrificeParameterization.SonicConductance  Cd=0.64  Cv_max=0.4  xT_Cv=0.7  Kv_max=0.3  xT_Kv=0.7  C_max=0.128 * (pi/4 * (0.003)^2) * 1000000 * 4/pi l/(s*bar)  B_crit_linear=0.41 + 0.272 * ((pi/4 * (0.003)^2)/(0.008) * 1)^0.25  m=0.5  T_ref_C=290 K  rho_ref_C=1.185 kg/m^3  leakage_fraction=(1e-12)/(pi/4 * (0.003)^2) * 1  smoothing_factor=0.7  B_lam=0.999  area=0.008 m^2  x0=0
      settings: InternalSimscapePortConfiguration="{\"Bottom\":[],\"Left\":[{\"id\":\"A\",\"label\":\"A\",\"type\":\"foundation.gas.gas\"},{\"id\":\"L\",\"label\":\"L\",\"type\":\"input\"}],\"Right\":[{\"id\":\"B\",\"label\":\"B\",\"type\":\"foundation.gas.gas\"}],\"Top\":[]}"
  opening1 : Subsystem
  p_atm : fl_lib/Gas/Elements/Reservoir (G)  pressure_spec=foundation.enum.pressure_spec.atmospheric  reservoir_pressure=p_atm Pa  reservoir_temperature=290 K  area_A=8e-4 m^2
  a : PMIOPort  Side=Left
  air : PMIOPort  Port=2  Side=Left
  guide_vane_opening : Outport
  wires:
  guide_vanes/1 -> opening1/1("guidevane ")
  opening1/1(guide vane opening) -> Simulink-PS Converter/1, guide_vane_opening/1
  connections:
  guide vanes air/LConn1 -- air/RConn1
  guide vanes air/LConn2 -- PS Switch/RConn1
  Simulink-PS Converter/RConn1 -- PS Switch/LConn2 -- a/RConn1
  PS Constant/RConn1 -- PS Switch/LConn1
  PS Constant1/RConn1 -- PS Switch/LConn3
  guide vanes air/RConn1 -- p_atm/LConn1

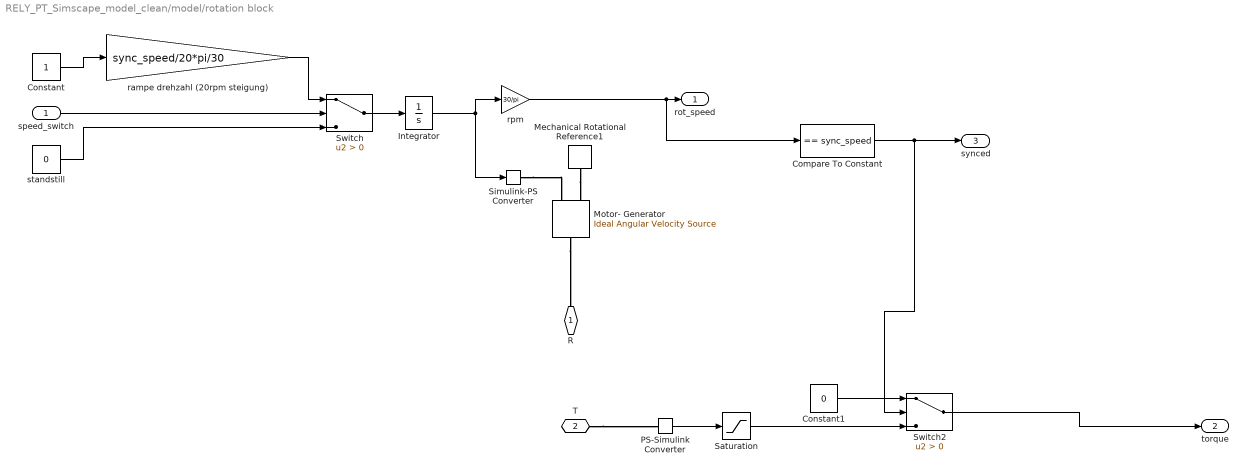
== system RELY_PT_Simscape_model_clean/model/rotation block ==
  speed_switch : Inport
  Compare To Constant : simulink/Logic and Bit Operations/Compare To Constant  relop===  const=sync_speed  OutDataTypeStr=boolean
  Constant : Constant
  Constant1 : Constant  Value=0
  Integrator : Integrator  LimitOutput=on  UpperSaturationLimit=sync_speed*pi/30  LowerSaturationLimit=0
  Mechanical Rotational Reference1 : fl_lib/Mechanical/Rotational Elements/Mechanical Rotational Reference
  Motor- Generator : fl_lib/Mechanical/Mechanical Sources/Ideal Angular Velocity Source
  PS-Simulink Converter : nesl_utility/PS-Simulink Converter  PhysicalDomain=network_engine_domain  SubClassName=ps_output  LeftPortType=input  RightPortType=output  PseudoPeriodic=off  Frequencies=[]  VectorFormat=inherit  Unit=inherit  AffineConversion=off
  Saturation : Saturate  UpperLimit=1000  LowerLimit=0
  Simulink-PS Converter : nesl_utility/Simulink-PS Converter  PhysicalDomain=network_engine_domain  SubClassName=ps_input  LeftPortType=input  RightPortType=output  PseudoPeriodic=off  Frequencies=[]  NoiseDistribution=none  NoiseParameters=[]  Unit=1  AffineConversion=off  FilteringAndDerivatives=filter  SimscapeFilterOrder=1  InputFilterTimeConstant=0.001  UdotUserProvided=0
  Switch : Switch  Criteria=u2 > Threshold  SaturateOnIntegerOverflow=off  InputSameDT=off
  Switch2 : Switch  Criteria=u2 > Threshold  SaturateOnIntegerOverflow=off  InputSameDT=off
  rampe drehzahl (20rpm steigung) : Gain  Gain=sync_speed/20*pi/30
  rpm : Gain  Gain=30/pi
  standstill : Constant  Value=0
  R : PMIOPort  Side=Right
  T : PMIOPort  Port=2  Side=Right
  rot_speed : Outport
  torque : Outport  Port=2
  synced : Outport  Port=3
  wires:
  rampe drehzahl (20rpm steigung)/1 -> Switch/1
  Switch/1 -> Integrator/1
  Constant/1 -> rampe drehzahl (20rpm steigung)/1
  speed_switch/1 -> Switch/2
  standstill/1 -> Switch/3
  Constant1/1 -> Switch2/1
  PS-Simulink Converter/1 -> Saturation/1
  Saturation/1 -> Switch2/3
  Compare To Constant/1 -> Switch2/2, synced/1
  Integrator/1 -> Simulink-PS Converter/1, rpm/1
  rpm/1 -> Compare To Constant/1, rot_speed/1
  Switch2/1 -> torque/1
  connections:
  Motor- Generator/LConn1 -- R/RConn1
  Mechanical Rotational Reference1/LConn1 -- Motor- Generator/RConn2
  Simulink-PS Converter/RConn1 -- Motor- Generator/RConn1
  T/RConn1 -- PS-Simulink Converter/LConn1

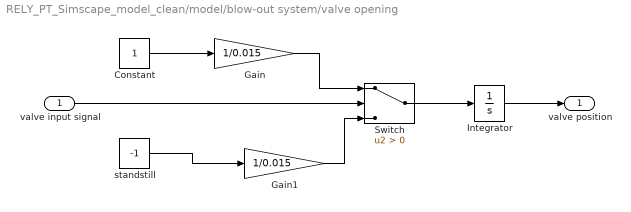
== system RELY_PT_Simscape_model_clean/model/blow-out system/valve opening ==
  valve input signal : Inport
  Constant : Constant
  Gain : Gain  Gain=1/0.015
  Gain1 : Gain  Gain=1/0.015
  Integrator : Integrator  LimitOutput=on  UpperSaturationLimit=1  LowerSaturationLimit=0
  Switch : Switch  Criteria=u2 > Threshold  SaturateOnIntegerOverflow=off  InputSameDT=off
  standstill : Constant  Value=-1
  valve position : Outport
  wires:
  valve input signal/1 -> Switch/2
  Switch/1 -> Integrator/1
  Gain/1 -> Switch/1
  Constant/1 -> Gain/1
  standstill/1 -> Gain1/1
  Integrator/1 -> valve position/1
  Gain1/1 -> Switch/3

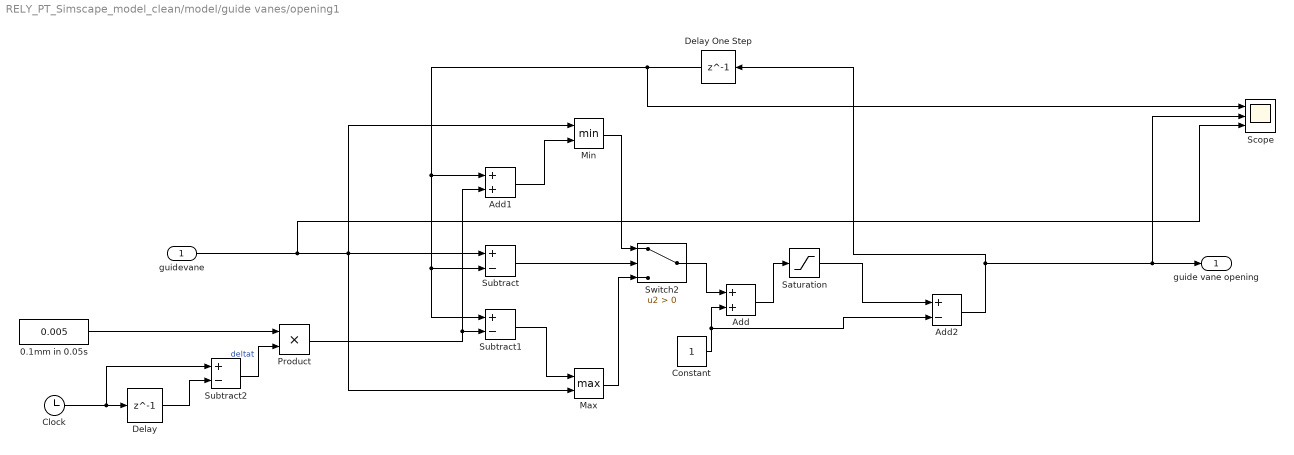
== system RELY_PT_Simscape_model_clean/model/guide vanes/opening1 ==
  "guidevane " : Inport
  0.1mm in 0.05s : Constant  Value=0.005
  Add : Sum
  Add1 : Sum
  Add2 : Sum  Inputs=+-
  Clock : Clock
  Constant : Constant
  Delay : Delay  DelayLength=1  InitialCondition=0
  Delay One Step : Delay  DelayLength=1  InitialCondition=a_max
  Max : MinMax  Function=max  Inputs=2
  Min : MinMax  Inputs=2
  Product : Product
  Saturation : Saturate  UpperLimit=a_max+1  LowerLimit=a_Spalt+1
  Scope : Scope  NumInputPorts=3
  Subtract : Sum  Inputs=+-
  Subtract1 : Sum  Inputs=+-
  Subtract2 : Sum  Inputs=+-
  Switch2 : Switch  Criteria=u2 > Threshold  OutMin=a_Spalt  SaturateOnIntegerOverflow=off  InputSameDT=off
  guide vane opening : Outport
  wires:
  "guidevane "/1 -> Scope/3, Subtract/1, Min/1, Max/2
  Min/1 -> Switch2/1
  Max/1 -> Switch2/3
  Delay One Step/1 -> Scope/1, Subtract1/1, Subtract/2, Add1/1
  Subtract1/1 -> Max/1
  0.1mm in 0.05s/1 -> Product/1
  Add1/1 -> Min/2
  Subtract/1 -> Switch2/2
  Clock/1 -> Delay/1, Subtract2/1
  Delay/1 -> Subtract2/2
  Subtract2/1 -> Product/2  "deltat"
  Product/1 -> Add1/2, Subtract1/2
  Add/1 -> Saturation/1
  Saturation/1 -> Add2/1
  Switch2/1 -> Add/1
  Constant/1 -> Add2/2, Add/2
  Add2/1 -> Delay One Step/1, Scope/2, guide vane opening/1

== matlab function RELY_PT_Simscape_model_clean/MATLAB Function ==
  data: N input double; air_valve output; guide_vanes output; speed_switch output; ball_valve output
function [air_valve, guide_vanes, speed_switch, ball_valve] = integer_to_array(N)
assert(isscalar(N), 'Action is no integer!');
guide_vane_vals = [0, 0.003, 0.006, 0.012, 0.018, 0.024, 0.03];
air_valve = mod(floor(N / (2*2*7)), 2);
guide_vanes = guide_vane_vals(mod(floor(N / (2*2)), 7) + 1);
speed_switch = mod(floor(N / 2), 2);
ball_valve = mod(N, 2);
end
